simulink model "gm_uz_pmsm_model_9ph_dq"  (R2021b)
settings: Solver=FixedStepAuto  StartTime=0.0  StopTime=0.8  RelTol=1e-3
undefined symbols (not defined in the file or in its folder): c, friction_coefficient, inertia, k_i_d, k_i_q, k_p_d, k_p_q, Kpd, L_d, L_q, L_x1, L_x2, L_x3, L_y1, L_y2, L_y3, L_zero, polepair, psi_pm, R_1, static_friction_torque, Tnd
libraries: hdlmdlgenlib x137, dspsigops x19, slpidlib x2, pid_lib x1, spsdq0toAlphaBetaZeroLib x1
(part 1 of 2)
settings Model: Creator=ts  LastModifiedBy=valen
settings SolverCC: AlgebraicLoopSolver=TrustRegion  AutoInsertRateTranBlk=on
settings DataIOCC: LimitDataPoints=on  SaveOutput=off  SaveTime=off
settings OptimizationCC: BlockReduction=off  ConditionallyExecuteInputs=off  DefaultParameterBehavior=Inlined  InheritOutputTypeSmallerThanSingle=on  LifeSpan=inf
settings DebuggingCC: AlgebraicLoopMsg=error  InheritedTsInSrcMsg=none  SingleTaskRateTransMsg=error  AllowSymbolicDim=off  StrictBusMsg=ErrorOnBusTreatedAsVector  SFUnexpectedBacktrackingDiag=warning  SFNoUnconditionalDefaultTransitionDiag=warning  SFExecutionAtInitializationDiag=none  SFMachineParentedDataDiag=warning  ArithmeticOperatorsInVariantConditions=warning
settings HardwareCC: ProdBitPerPointer=32  ProdBitPerSizeT=32  ProdBitPerPtrDiffT=32  ProdLargestAtomicFloat=None  ProdIntDivRoundTo=Undefined  ProdEndianess=Unspecified  ProdWordSize=32  ProdHWDeviceType=ASIC/FPGA->ASIC/FPGA  ProdEqTarget=off
settings SFSimCC: SimUseLocalCustomCode=off  CustomCodeUndefinedFunction=UseInterfaceOnly
settings RTWCC: RTWUseLocalCustomCode=off
settings CodeAppCC: StateflowObjectComments=on
settings GRTTargetCC: TargetLangStandard=C89/C90 (ANSI)
settings ConfigComp: CovScope=ReferencedModels  CovMetricSettings=dw  CovSaveCumulativeToWorkspaceVar=on  CovSaveSingleToWorkspaceVar=on  CovExternalEMLEnable=off  CovSFcnEnable=off

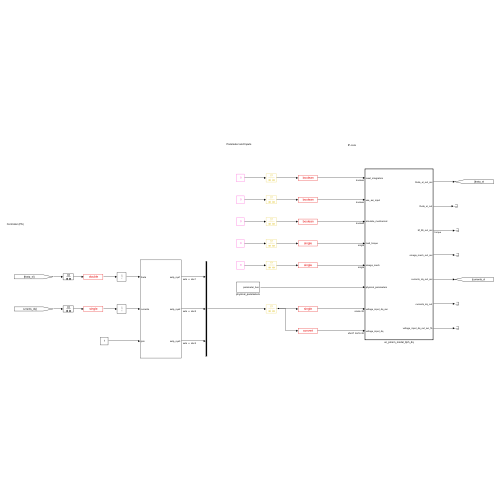
[thumbnail: Simulink's stored preview of the top-level diagram]
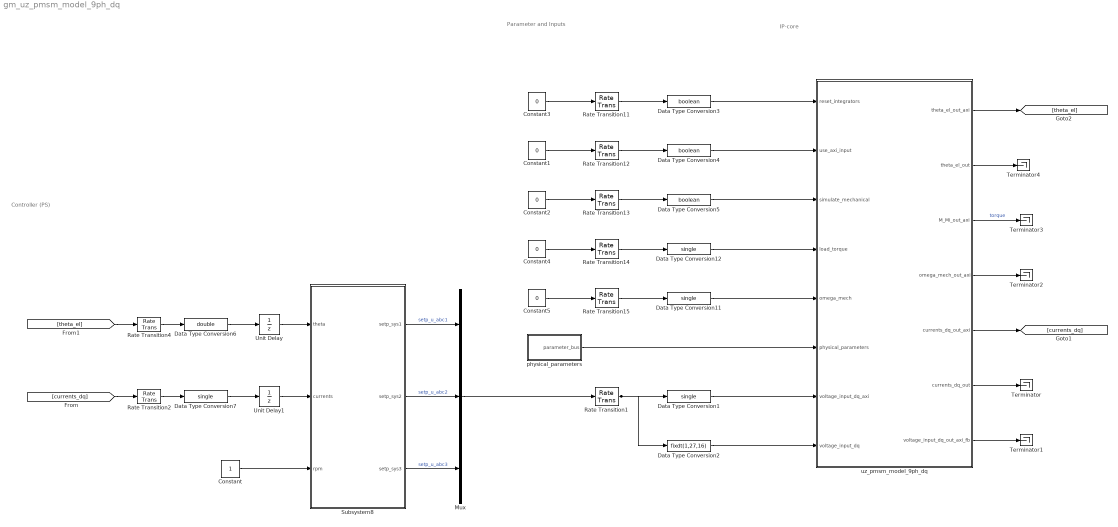
== system gm_uz_pmsm_model_9ph_dq ==
  note: IP-core
  note: Parameter and Inputs
  note: Controller (PS)
  Constant : Constant
  Constant{1..5} (5 alike) : Constant  Value=0
  Data Type Conversion{1,7,11..12} (4 alike) : DataTypeConversion  OutDataTypeStr=single
  Data Type Conversion2 : DataTypeConversion  OutDataTypeStr=fixdt(1,27,16)
  Data Type Conversion3 : DataTypeConversion  OutDataTypeStr=boolean
  Data Type Conversion4 : DataTypeConversion  OutDataTypeStr=boolean
  Data Type Conversion5 : DataTypeConversion  OutDataTypeStr=boolean
  Data Type Conversion6 : DataTypeConversion  OutDataTypeStr=double
  Mux : Mux  Inputs=3
  Rate Transition{1,11..15} (6 alike) : RateTransition  OutPortSampleTime=ts_pmsm
  Rate Transition2 : RateTransition  OutPortSampleTime=ts_isr
  Rate Transition4 : RateTransition  OutPortSampleTime=ts_isr
  Subsystem8 : Subsystem
  Terminator{,1..4} (5 alike) : Terminator
  Unit Delay : UnitDelay  SampleTime=-1  HasFrameUpgradeWarning=on
  Unit Delay1 : UnitDelay  SampleTime=-1  HasFrameUpgradeWarning=on
  physical_parameters : Subsystem
  uz_pmsm_model_9ph_dq : Subsystem  TreatAsAtomicUnit=on
  wires:
  Constant/1 -> Subsystem8/3(rpm)
  uz_pmsm_model_9ph_dq/2(theta_el_out) -> Terminator4/1
  uz_pmsm_model_9ph_dq/3(M_Mi_out_axi) -> Terminator3/1  "torque"
  uz_pmsm_model_9ph_dq/4(omega_mech_out_axi) -> Terminator2/1
  uz_pmsm_model_9ph_dq/7(voltage_input_dq_out_axi_fb) -> Terminator1/1
  uz_pmsm_model_9ph_dq/6(currents_dq_out) -> Terminator/1
  uz_pmsm_model_9ph_dq/5(currents_dq_out_axi) -> [currents_dq]
  uz_pmsm_model_9ph_dq/1(theta_el_out_axi) -> [theta_el]
  [currents_dq] -> Rate Transition2/1
  Data Type Conversion7/1 -> Unit Delay1/1
  Rate Transition2/1 -> Data Type Conversion7/1
  Unit Delay1/1 -> Subsystem8/2(currents)
  Unit Delay/1 -> Subsystem8/1(theta)
  Mux/1 -> Rate Transition1/1
  Data Type Conversion2/1 -> uz_pmsm_model_9ph_dq/8(voltage_input_dq)
  Data Type Conversion1/1 -> uz_pmsm_model_9ph_dq/7(voltage_input_dq_axi)
  Rate Transition1/1 -> Data Type Conversion1/1, Data Type Conversion2/1
  Subsystem8/1(setp_sys1) -> Mux/1  "setp_u_abc1"
  Subsystem8/2(setp_sys2) -> Mux/2  "setp_u_abc2"
  Subsystem8/3(setp_sys3) -> Mux/3  "setp_u_abc3"
  physical_parameters/1(parameter_bus) -> uz_pmsm_model_9ph_dq/6(physical_parameters)
  Constant4/1 -> Rate Transition14/1
  Constant5/1 -> Rate Transition15/1
  Data Type Conversion11/1 -> uz_pmsm_model_9ph_dq/5(omega_mech)
  Data Type Conversion12/1 -> uz_pmsm_model_9ph_dq/4(load_torque)
  Rate Transition14/1 -> Data Type Conversion12/1
  Rate Transition15/1 -> Data Type Conversion11/1
  Data Type Conversion5/1 -> uz_pmsm_model_9ph_dq/3(simulate_mechanical)
  Rate Transition13/1 -> Data Type Conversion5/1
  Constant2/1 -> Rate Transition13/1
  Constant1/1 -> Rate Transition12/1
  Rate Transition12/1 -> Data Type Conversion4/1
  Data Type Conversion4/1 -> uz_pmsm_model_9ph_dq/2(use_axi_input)
  Data Type Conversion3/1 -> uz_pmsm_model_9ph_dq/1(reset_integrators)
  Rate Transition11/1 -> Data Type Conversion3/1
  Constant3/1 -> Rate Transition11/1
  Rate Transition4/1 -> Data Type Conversion6/1
  Data Type Conversion6/1 -> Unit Delay/1
  [theta_el] -> Rate Transition4/1

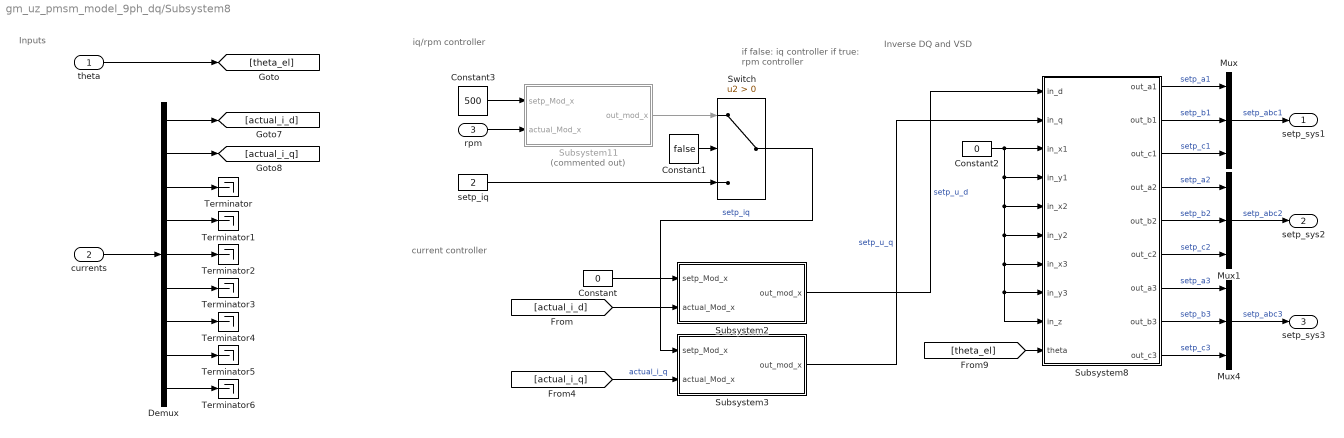
== system gm_uz_pmsm_model_9ph_dq/Subsystem8 ==
  note: Inverse DQ and VSD
  note: if false: iq controller
      | if true: rpm controller
  note: iq/rpm controller
  note: current controller
  note: Inputs
  theta : Inport
  currents : Inport  Port=2
  rpm : Inport  Port=3
  Constant : Constant  Value=0
  Constant1 : Constant  Value=false
  Constant2 : Constant  Value=0
  Constant3 : Constant  Value=500
  Demux : Demux  Outputs=9
  Mux : Mux  Inputs=3
  Mux1 : Mux  Inputs=3
  Mux4 : Mux  Inputs=3
  Subsystem11 : Subsystem  Commented=on
  Subsystem2 : Subsystem
  Subsystem3 : Subsystem
  Subsystem8 : Subsystem
  Switch : Switch  Criteria=u2 > Threshold
  Terminator{,1..6} (7 alike) : Terminator
  setp_iq : Constant  Value=2
  setp_sys1 : Outport
  setp_sys2 : Outport  Port=2
  setp_sys3 : Outport  Port=3
  wires:
  Demux/9 -> Terminator6/1
  Demux/6 -> Terminator3/1
  Demux/7 -> Terminator4/1
  Demux/8 -> Terminator5/1
  Demux/5 -> Terminator2/1
  Demux/4 -> Terminator1/1
  Demux/3 -> Terminator/1
  Demux/2 -> [actual_i_q]
  Demux/1 -> [actual_i_d]
  currents/1 -> Demux/1
  Subsystem2/1(out_mod_x) -> Subsystem8/1(in_d)  "setp_u_d"
  Subsystem3/1(out_mod_x) -> Subsystem8/2(in_q)  "setp_u_q"
  Constant3/1 -> Subsystem11/1(setp_Mod_x)
  setp_iq/1 -> Switch/3
  Constant1/1 -> Switch/2
  Switch/1 -> Subsystem3/1(setp_Mod_x)  "setp_iq"
  Subsystem11/1(out_mod_x) -> Switch/1
  Constant2/1 -> Subsystem8/4(in_y1), Subsystem8/5(in_x2), Subsystem8/6(in_y2), Subsystem8/7(in_x3), Subsystem8/9(in_z), Subsystem8/8(in_y3), Subsystem8/3(in_x1)
  rpm/1 -> Subsystem11/2(actual_Mod_x)
  Subsystem8/9(out_c3) -> Mux4/3  "setp_c3"
  Subsystem8/8(out_b3) -> Mux4/2  "setp_b3"
  Subsystem8/7(out_a3) -> Mux4/1  "setp_a3"
  Mux4/1 -> setp_sys3/1  "setp_abc3"
  Subsystem8/4(out_a2) -> Mux1/1  "setp_a2"
  Subsystem8/5(out_b2) -> Mux1/2  "setp_b2"
  Subsystem8/6(out_c2) -> Mux1/3  "setp_c2"
  Mux1/1 -> setp_sys2/1  "setp_abc2"
  Mux/1 -> setp_sys1/1  "setp_abc1"
  theta/1 -> [theta_el]
  [actual_i_q] -> Subsystem3/2(actual_Mod_x)  "actual_i_q"
  Constant/1 -> Subsystem2/1(setp_Mod_x)
  [actual_i_d] -> Subsystem2/2(actual_Mod_x)
  Subsystem8/3(out_c1) -> Mux/3  "setp_c1"
  Subsystem8/2(out_b1) -> Mux/2  "setp_b1"
  [theta_el] -> Subsystem8/10(theta)
  Subsystem8/1(out_a1) -> Mux/1  "setp_a1"

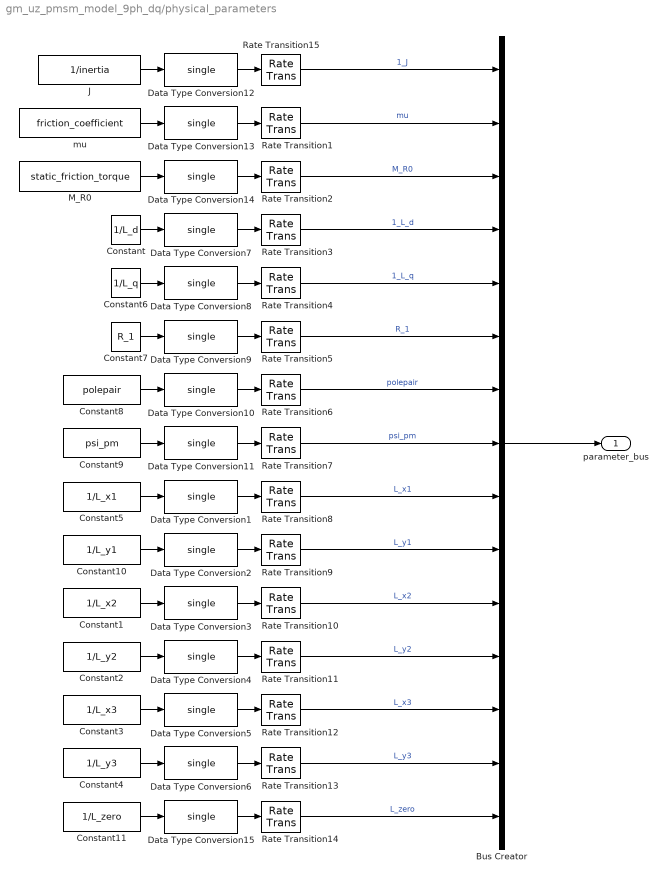
== system gm_uz_pmsm_model_9ph_dq/physical_parameters ==
  Bus Creator : BusCreator  Inputs=15
  Constant : Constant  Value=1/L_d
  Constant1 : Constant  Value=1/L_x2
  Constant10 : Constant  Value=1/L_y1
  Constant11 : Constant  Value=1/L_zero
  Constant2 : Constant  Value=1/L_y2
  Constant3 : Constant  Value=1/L_x3
  Constant4 : Constant  Value=1/L_y3
  Constant5 : Constant  Value=1/L_x1
  Constant6 : Constant  Value=1/L_q
  Constant7 : Constant  Value=R_1
  Constant8 : Constant  Value=polepair
  Constant9 : Constant  Value=psi_pm
  Data Type Conversion{1..15} (15 alike) : DataTypeConversion  OutDataTypeStr=single
  J : Constant  Value=1/inertia
  M_R0 : Constant  Value=static_friction_torque
  Rate Transition{1..15} (15 alike) : RateTransition  OutPortSampleTime=ts_pmsm
  mu : Constant  Value=friction_coefficient
  parameter_bus : Outport
  wires:
  Constant10/1 -> Data Type Conversion2/1
  Constant5/1 -> Data Type Conversion1/1
  Constant1/1 -> Data Type Conversion3/1
  Constant2/1 -> Data Type Conversion4/1
  Constant3/1 -> Data Type Conversion5/1
  Constant4/1 -> Data Type Conversion6/1
  Rate Transition9/1 -> Bus Creator/10  "L_y1"
  Rate Transition10/1 -> Bus Creator/11  "L_x2"
  Rate Transition11/1 -> Bus Creator/12  "L_y2"
  Rate Transition12/1 -> Bus Creator/13  "L_x3"
  Rate Transition13/1 -> Bus Creator/14  "L_y3"
  Rate Transition14/1 -> Bus Creator/15  "L_zero"
  Rate Transition8/1 -> Bus Creator/9  "L_x1"
  Data Type Conversion15/1 -> Rate Transition14/1
  Constant11/1 -> Data Type Conversion15/1
  Data Type Conversion6/1 -> Rate Transition13/1
  Data Type Conversion5/1 -> Rate Transition12/1
  Data Type Conversion4/1 -> Rate Transition11/1
  Data Type Conversion3/1 -> Rate Transition10/1
  Data Type Conversion2/1 -> Rate Transition9/1
  Data Type Conversion1/1 -> Rate Transition8/1
  Constant/1 -> Data Type Conversion7/1
  Constant9/1 -> Data Type Conversion11/1
  Constant7/1 -> Data Type Conversion9/1
  Data Type Conversion13/1 -> Rate Transition1/1
  Rate Transition4/1 -> Bus Creator/5  "1_L_q"
  M_R0/1 -> Data Type Conversion14/1
  mu/1 -> Data Type Conversion13/1
  Data Type Conversion10/1 -> Rate Transition6/1
  Data Type Conversion8/1 -> Rate Transition4/1
  J/1 -> Data Type Conversion12/1
  Rate Transition3/1 -> Bus Creator/4  "1_L_d"
  Constant6/1 -> Data Type Conversion8/1
  Rate Transition1/1 -> Bus Creator/2  "mu"
  Data Type Conversion9/1 -> Rate Transition5/1
  Constant8/1 -> Data Type Conversion10/1
  Data Type Conversion11/1 -> Rate Transition7/1
  Bus Creator/1 -> parameter_bus/1
  Rate Transition6/1 -> Bus Creator/7  "polepair"
  Rate Transition15/1 -> Bus Creator/1  "1_J"
  Rate Transition5/1 -> Bus Creator/6  "R_1"
  Data Type Conversion14/1 -> Rate Transition2/1
  Rate Transition7/1 -> Bus Creator/8  "psi_pm"
  Rate Transition2/1 -> Bus Creator/3  "M_R0"
  Data Type Conversion7/1 -> Rate Transition3/1
  Data Type Conversion12/1 -> Rate Transition15/1

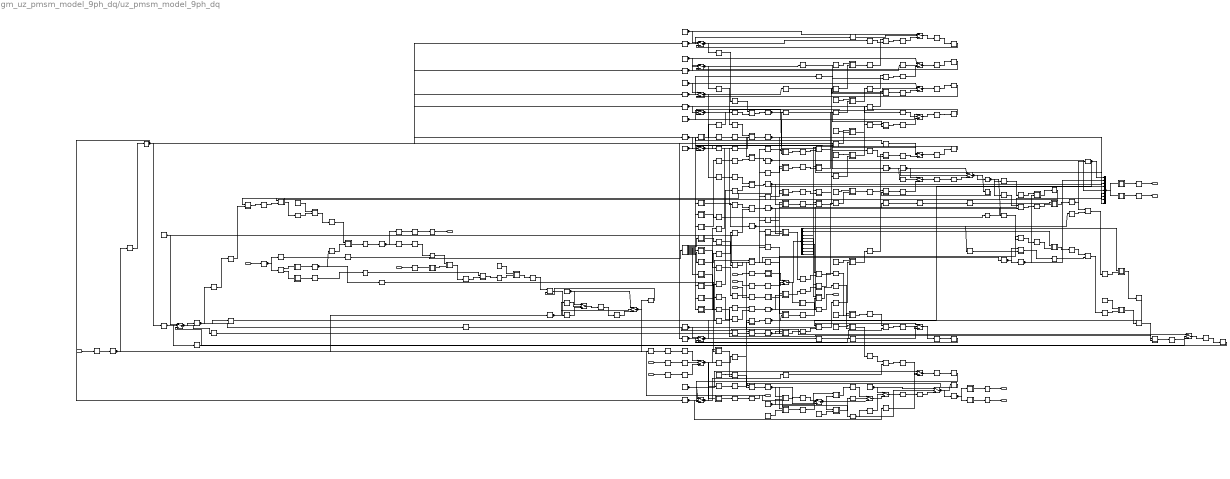
== system gm_uz_pmsm_model_9ph_dq/uz_pmsm_model_9ph_dq ==
  note: https://de.mathworks.com/help/releases/R2021a/hdlcoder/ug/troubleshoot-generate-implementation-model-from-simscape-pmsm.html?searchHighlight=troubleshoot-generate-implementation-model-from-simscape-pmsm&s_tid=doc_srchtitle
  note: load torque negative!!!
  note: zero equation
  note: y2 equation
  note: x2 equation
  note: y1 equation
  note: x1 equation
  note: o2 equation
  note: DQ equations
  note: o1 equation
  note: Inputs
  note: Mechanical and output
  note: PMSM electric and magentic
  note: This signal introduces an algebraic loop if simulate_mechanical is true!
  note: Input
  reset_integrators : Inport  OutDataTypeStr=boolean  PortDimensions=1  SampleTime=1e-06
  use_axi_input : Inport  Port=2  OutDataTypeStr=boolean  PortDimensions=1  SampleTime=1e-06
  simulate_mechanical : Inport  Port=3  OutDataTypeStr=boolean  PortDimensions=1  SampleTime=1e-06
  load_torque : Inport  Port=4  OutDataTypeStr=single  PortDimensions=1  SampleTime=1e-06
  omega_mech : Inport  Port=5  OutDataTypeStr=single  PortDimensions=1  SampleTime=1e-06
  physical_parameters : Inport  Port=6  SampleTime=1e-06
  voltage_input_dq_axi : Inport  Port=7  OutDataTypeStr=single  PortDimensions=[9]  SampleTime=1e-06
  voltage_input_dq : Inport  Port=8  OutDataTypeStr=fixdt(1, 27, 16)  PortDimensions=[9]  SampleTime=1e-06
  Add : Subsystem
      mask Display: disp('NFP\nadd');
  Add1 : Subsystem
      mask Display: disp('NFP\nadd');
  Add1_outbuff : hdlmdlgenlib/Buffer
      settings: SourceProductBaseCode=SL
  Add2 : Subsystem
      mask Display: disp('NFP\nadd');
  Add2_outbuff : hdlmdlgenlib/Buffer
      settings: SourceProductBaseCode=SL
  Add3 : Subsystem
      mask Display: disp('NFP\nadd');
  Add3_outbuff : hdlmdlgenlib/Buffer
      settings: SourceProductBaseCode=SL
  Add4 : Subsystem
      mask Display: disp('NFP\nadd');
  Add4_outbuff : hdlmdlgenlib/Buffer
      settings: SourceProductBaseCode=SL
  Add5 : Subsystem
      mask Display: disp('NFP\nadd');
  Add5_outbuff : hdlmdlgenlib/Buffer
      settings: SourceProductBaseCode=SL
  Add6 : Subsystem
      mask Display: disp('NFP\nadd');
  Add6_outbuff : hdlmdlgenlib/Buffer
      settings: SourceProductBaseCode=SL
  Add_outbuff : hdlmdlgenlib/Buffer
      settings: SourceProductBaseCode=SL
  Compare To Constant1_const : Constant  Value=double(-3.1415927410125732)  OutDataTypeStr=double  SampleTime=1e-08
  Compare To Constant1_relop : Subsystem
      mask Display: disp('NFP\nrelop');
  Compare To Constant1_relop_outbuff : hdlmdlgenlib/Buffer
      settings: SourceProductBaseCode=SL
  Compare To Constant_const : Constant  Value=double(3.1415927410125732)  OutDataTypeStr=double  SampleTime=1e-08
  Compare To Constant_relop : Subsystem
      mask Display: disp('NFP\nrelop');
  Compare To Constant_relop_outbuff : hdlmdlgenlib/Buffer
      settings: SourceProductBaseCode=SL
  Constant : Constant  Value=double(6.283185307179586)  OutDataTypeStr=double  SampleTime=1e-08
  Data Type Conversion1 : Subsystem
      mask Display: disp('NFP\nconv');
  Data Type Conversion10 : Subsystem
      mask Display: disp('NFP\nconv');
  Data Type Conversion101 : Subsystem
      mask Display: disp('NFP\nconv');
  Data Type Conversion11 : Subsystem
      mask Display: disp('NFP\nconv');
  Data Type Conversion111 : Subsystem
      mask Display: disp('NFP\nconv');
  Data Type Conversion12 : Subsystem
      mask Display: disp('NFP\nconv');
  Data Type Conversion121 : Subsystem
      mask Display: disp('NFP\nconv');
  Data Type Conversion13 : Subsystem
      mask Display: disp('NFP\nconv');
  Data Type Conversion14 : Subsystem
      mask Display: disp('NFP\nconv');
  Data Type Conversion15 : Subsystem
      mask Display: disp('NFP\nconv');
  Data Type Conversion2 : Subsystem
      mask Display: disp('NFP\nconv');
  Data Type Conversion21 : Subsystem
      mask Display: disp('NFP\nconv');
  Data Type Conversion3 : Subsystem
      mask Display: disp('NFP\nconv');
  Data Type Conversion31 : Subsystem
      mask Display: disp('NFP\nconv');
  Data Type Conversion4 : Subsystem
      mask Display: disp('NFP\nconv');
  Data Type Conversion41 : Subsystem
      mask Display: disp('NFP\nconv');
  Data Type Conversion5 : Subsystem
      mask Display: disp('NFP\nconv');
  Data Type Conversion51 : Subsystem
      mask Display: disp('NFP\nconv');
  Data Type Conversion6 : Subsystem
      mask Display: disp('NFP\nconv');
  Data Type Conversion61 : Subsystem
      mask Display: disp('NFP\nconv');
  Data Type Conversion7 : Subsystem
      mask Display: disp('NFP\nconv');
  Data Type Conversion71 : Subsystem
      mask Display: disp('NFP\nconv');
  Data Type Conversion8 : Subsystem
      mask Display: disp('NFP\nconv');
  Data Type Conversion81 : Subsystem
      mask Display: disp('NFP\nconv');
  Data Type Conversion9 : Subsystem
      mask Display: disp('NFP\nconv');
  Delay : RateTransition  OutPortSampleTimeOpt=Multiple of input port sample time  OutPortSampleTimeMultiple=100
  Delay1 : RateTransition  OutPortSampleTimeOpt=Multiple of input port sample time  OutPortSampleTimeMultiple=100
  Delay1_lowered{,1..10} (11 alike) : RateTransition  OutPortSampleTimeOpt=Multiple of input port sample time  OutPortSampleTimeMultiple=100
  Delay2 : RateTransition  OutPortSampleTimeOpt=Multiple of input port sample time  OutPortSampleTimeMultiple=100
  Divide : Subsystem
      mask Display: disp('NFP\nmul');
  Divide1 : Subsystem
      mask Display: disp('NFP\nmul');
  Divide10 : Subsystem
      mask Display: disp('NFP\nmul');
  Divide10_outbuff : hdlmdlgenlib/Buffer
      settings: SourceProductBaseCode=SL
  Divide11 : Subsystem
      mask Display: disp('NFP\nmul');
  Divide11_outbuff : hdlmdlgenlib/Buffer
      settings: SourceProductBaseCode=SL
  Divide12 : Subsystem
      mask Display: disp('NFP\nmul');
  Divide12_outbuff : hdlmdlgenlib/Buffer
      settings: SourceProductBaseCode=SL
  Divide13 : Subsystem
      mask Display: disp('NFP\nmul');
  Divide13_outbuff : hdlmdlgenlib/Buffer
      settings: SourceProductBaseCode=SL
  Divide1_outbuff : hdlmdlgenlib/Buffer
      settings: SourceProductBaseCode=SL
  Divide2 : Subsystem
      mask Display: disp('NFP\nmul');
  Divide2_outbuff : hdlmdlgenlib/Buffer
      settings: SourceProductBaseCode=SL
  Divide3 : Subsystem
      mask Display: disp('NFP\nmul');
  Divide3_outbuff : hdlmdlgenlib/Buffer
      settings: SourceProductBaseCode=SL
  Divide4 : Subsystem
      mask Display: disp('NFP\nmul');
  Divide4_outbuff : hdlmdlgenlib/Buffer
      settings: SourceProductBaseCode=SL
  Divide5 : Subsystem
      mask Display: disp('NFP\nmul');
  Divide5_outbuff : hdlmdlgenlib/Buffer
      settings: SourceProductBaseCode=SL
  Divide6 : Subsystem
      mask Display: disp('NFP\nmul');
  Divide6_outbuff : hdlmdlgenlib/Buffer
      settings: SourceProductBaseCode=SL
  Divide7 : Subsystem
      mask Display: disp('NFP\nmul');
  Divide7_outbuff : hdlmdlgenlib/Buffer
      settings: SourceProductBaseCode=SL
  Divide8 : Subsystem
      mask Display: disp('NFP\nmul');
  Divide8_outbuff : hdlmdlgenlib/Buffer
      settings: SourceProductBaseCode=SL
  Divide9 : Subsystem
      mask Display: disp('NFP\nmul');
  Divide9_outbuff : hdlmdlgenlib/Buffer
      settings: SourceProductBaseCode=SL
  Divide_outbuff : hdlmdlgenlib/Buffer
      settings: SourceProductBaseCode=SL
  Factor : Subsystem
      mask Display: disp('NFP\nmul');
  Factor_const : Constant  Value=double(4.5)  OutDataTypeStr=double  SampleTime=1e-08
  Factor_outbuff : hdlmdlgenlib/Buffer
      settings: SourceProductBaseCode=SL
  From{,1..27,30..32,41,51,61,71,91,121} (37 alike) : hdlmdlgenlib/Buffer
      settings: SourceProductBaseCode=SL
  Gain : Subsystem
      mask Display: disp('NFP\nmul');
  Gain1 : Subsystem
      mask Display: disp('NFP\nmul');
  Gain10 : Subsystem
      mask Display: disp('NFP\nmul');
  Gain2 : Subsystem
      mask Display: disp('NFP\nmul');
  Gain3 : Subsystem
      mask Display: disp('NFP\nmul');
  Gain4 : Subsystem
      mask Display: disp('NFP\nmul');
  Gain5 : Subsystem
      mask Display: disp('NFP\nmul');
  Gain6 : Subsystem
      mask Display: disp('NFP\nmul');
  Gain7 : Subsystem
      mask Display: disp('NFP\nmul');
  Gain8 : Subsystem
      mask Display: disp('NFP\nmul');
  Gain9 : Subsystem
      mask Display: disp('NFP\nmul');
  Gain_const{,1..10} (11 alike) : Constant  Value=double(1e-06)  OutDataTypeStr=double  SampleTime=1e-08
  Gain_outbuff{,1..9} (10 alike) : hdlmdlgenlib/Buffer
      settings: SourceProductBaseCode=SL
  Goto{1..4,9..16,32..36,361} (18 alike) : hdlmdlgenlib/Buffer
      settings: SourceProductBaseCode=SL
  Initial_Val{,1..10} (11 alike) : Constant  Value=double(0)  OutDataTypeStr=double  SampleTime=1e-08
  M_Mi : hdlmdlgenlib/Buffer
      settings: SourceProductBaseCode=SL
  Product : Subsystem
      mask Display: disp('NFP\nmul');
  Product1 : Subsystem
      mask Display: disp('NFP\nmul');
  Product10 : Subsystem
      mask Display: disp('NFP\nmul');
  Product10_outbuff : hdlmdlgenlib/Buffer
      settings: SourceProductBaseCode=SL
  Product11 : Subsystem
      mask Display: disp('NFP\nmul');
  Product11_outbuff : hdlmdlgenlib/Buffer
      settings: SourceProductBaseCode=SL
  Product1_outbuff : hdlmdlgenlib/Buffer
      settings: SourceProductBaseCode=SL
  Product2 : Subsystem
      mask Display: disp('NFP\nmul');
  Product21 : Subsystem
      mask Display: disp('NFP\nmul');
  Product2_outbuff : hdlmdlgenlib/Buffer
      settings: SourceProductBaseCode=SL
  Product3 : Subsystem
      mask Display: disp('NFP\nmul');
  Product3_outbuff : hdlmdlgenlib/Buffer
      settings: SourceProductBaseCode=SL
  Product5 : Subsystem
      mask Display: disp('NFP\nmul');
  Product5_outbuff : hdlmdlgenlib/Buffer
      settings: SourceProductBaseCode=SL
  Product6 : Subsystem
      mask Display: disp('NFP\nmul');
  Product6_outbuff : hdlmdlgenlib/Buffer
      settings: SourceProductBaseCode=SL
  Product7 : Subsystem
      mask Display: disp('NFP\nmul');
  Product7_outbuff : hdlmdlgenlib/Buffer
      settings: SourceProductBaseCode=SL
  Product8 : Subsystem
      mask Display: disp('NFP\nmul');
  Product8_outbuff : hdlmdlgenlib/Buffer
      settings: SourceProductBaseCode=SL
  Product9 : Subsystem
      mask Display: disp('NFP\nmul');
  Product9_outbuff : hdlmdlgenlib/Buffer
      settings: SourceProductBaseCode=SL
  Product_outbuff : hdlmdlgenlib/Buffer
      settings: SourceProductBaseCode=SL
  Sum : Subsystem
      mask Display: disp('NFP\nadd');
  Sum1 : Subsystem
      mask Display: disp('NFP\nadd');
  Sum11 : Subsystem
      mask Display: disp('NFP\nadd');
  Sum1_outbuff : hdlmdlgenlib/Buffer
      settings: SourceProductBaseCode=SL
  Sum1_outbuff1 : hdlmdlgenlib/Buffer
      settings: SourceProductBaseCode=SL
  Sum1_stage2 : Subsystem
      mask Display: disp('NFP\nadd');
  Sum1_stage2_outbuff : hdlmdlgenlib/Buffer
      settings: SourceProductBaseCode=SL
  Sum1_stage3 : Subsystem
      mask Display: disp('NFP\nadd');
  Sum1_stage3_outbuff : hdlmdlgenlib/Buffer
      settings: SourceProductBaseCode=SL
  Sum2 : Subsystem
      mask Display: disp('NFP\nadd');
  Sum21 : Subsystem
      mask Display: disp('NFP\nadd');
  Sum2_outbuff : hdlmdlgenlib/Buffer
      settings: SourceProductBaseCode=SL
  Sum2_outbuff1 : hdlmdlgenlib/Buffer
      settings: SourceProductBaseCode=SL
  Sum3 : Subsystem
      mask Display: disp('NFP\nadd');
  Sum31 : Subsystem
      mask Display: disp('NFP\nadd');
  Sum310 : Subsystem
      mask Display: disp('NFP\nadd');
  Sum32 : Subsystem
      mask Display: disp('NFP\nadd');
  Sum33 : Subsystem
      mask Display: disp('NFP\nadd');
  Sum34 : Subsystem
      mask Display: disp('NFP\nadd');
  Sum35 : Subsystem
      mask Display: disp('NFP\nadd');
  Sum36 : Subsystem
      mask Display: disp('NFP\nadd');
  Sum37 : Subsystem
      mask Display: disp('NFP\nadd');
  Sum38 : Subsystem
      mask Display: disp('NFP\nadd');
  Sum39 : Subsystem
      mask Display: disp('NFP\nadd');
  Sum3_outbuff{,1..10} (11 alike) : hdlmdlgenlib/Buffer
      settings: SourceProductBaseCode=SL
  Sum_outbuff : hdlmdlgenlib/Buffer
      settings: SourceProductBaseCode=SL
  Sum_stage2 : Subsystem
      mask Display: disp('NFP\nadd');
  Sum_stage2_outbuff : hdlmdlgenlib/Buffer
      settings: SourceProductBaseCode=SL
  Sum_stage3 : Subsystem
      mask Display: disp('NFP\nadd');
  Sum_stage3_outbuff : hdlmdlgenlib/Buffer
      settings: SourceProductBaseCode=SL
  Switch{,1..2,11} (4 alike) : Switch  Criteria=u2 ~= 0  Threshold=double(0)  OutDataTypeStr=double  SampleTime=1e-08
  bus_selector : BusSelector  OutputSignals=1_L_d,1_L_q,R_1,polepair,psi_pm,L_x1,L_y1,L_x2,L_y2,L_x3,L_y3,L_zero
  bus_selector1 : BusSelector  OutputSignals=polepair,1_J
  delayMatch{,1..38} (39 alike) : Delay  DelayLength=double(1)  InitialCondition=0  SampleTime=1e-08
  delayMatch39 : Delay  DelayLength=double(1)  InitialCondition=0  SampleTime=1e-06
  delayMatch40 : Delay  DelayLength=double(1)  InitialCondition=0  SampleTime=1e-06
  i_d : hdlmdlgenlib/Buffer
      settings: SourceProductBaseCode=SL
  i_q : hdlmdlgenlib/Buffer
      settings: SourceProductBaseCode=SL
  in0_repeat : dspsigops/Repeat  N=double(100)  RateOptions=Allow multirate processing  ic=0  mode=Unused parameter value
  in10_repeat : dspsigops/Repeat  N=double(100)  RateOptions=Allow multirate processing  ic=0  mode=Unused parameter value
  in11_repeat : dspsigops/Repeat  N=double(100)  RateOptions=Allow multirate processing  ic=0  mode=Unused parameter value
  in12_repeat : dspsigops/Repeat  N=double(100)  RateOptions=Allow multirate processing  ic=0  mode=Unused parameter value
  in13_repeat : RateTransition  Integrity=off  Deterministic=off  OutPortSampleTimeOpt=Multiple of input port sample time  OutPortSampleTimeMultiple=1/100
  in14_repeat : dspsigops/Repeat  N=double(100)  RateOptions=Allow multirate processing  ic=0  mode=Unused parameter value
  in15_repeat : dspsigops/Repeat  N=double(100)  RateOptions=Allow multirate processing  ic=0  mode=Unused parameter value
  in16_repeat : dspsigops/Repeat  N=double(100)  RateOptions=Allow multirate processing  ic=0  mode=Unused parameter value
  in17_repeat : dspsigops/Repeat  N=double(100)  RateOptions=Allow multirate processing  ic=0  mode=Unused parameter value
  in18_repeat : dspsigops/Repeat  N=double(100)  RateOptions=Allow multirate processing  ic=0  mode=Unused parameter value
  in19_repeat : dspsigops/Repeat  N=double(100)  RateOptions=Allow multirate processing  ic=0  mode=Unused parameter value
  in1_repeat : dspsigops/Repeat  N=double(100)  RateOptions=Allow multirate processing  ic=0  mode=Unused parameter value
  in2_repeat : dspsigops/Repeat  N=double(100)  RateOptions=Allow multirate processing  ic=0  mode=Unused parameter value
  in3_repeat : dspsigops/Repeat  N=double(100)  RateOptions=Allow multirate processing  ic=0  mode=Unused parameter value
  in4_repeat : dspsigops/Repeat  N=double(100)  RateOptions=Allow multirate processing  ic=0  mode=Unused parameter value
  in5_repeat : dspsigops/Repeat  N=double(100)  RateOptions=Allow multirate processing  ic=0  mode=Unused parameter value
  in6_repeat : dspsigops/Repeat  N=double(100)  RateOptions=Allow multirate processing  ic=0  mode=Unused parameter value
  in7_repeat : dspsigops/Repeat  N=double(100)  RateOptions=Allow multirate processing  ic=0  mode=Unused parameter value
  in8_repeat : dspsigops/Repeat  N=double(100)  RateOptions=Allow multirate processing  ic=0  mode=Unused parameter value
  in9_repeat : dspsigops/Repeat  N=double(100)  RateOptions=Allow multirate processing  ic=0  mode=Unused parameter value
  integrator_out1 : hdlmdlgenlib/Buffer
      settings: SourceProductBaseCode=SL
  mechanical_system_out1 : hdlmdlgenlib/Buffer
      settings: SourceProductBaseCode=SL
  mux : Mux  Inputs=9
  pmsm_out1 : hdlmdlgenlib/Buffer
      settings: SourceProductBaseCode=SL
  pmsm_out2 : hdlmdlgenlib/Buffer
      settings: SourceProductBaseCode=SL
  psi_{,1..6} (7 alike) : hdlmdlgenlib/Buffer
      settings: SourceProductBaseCode=SL
  psi_d : hdlmdlgenlib/Buffer
      settings: SourceProductBaseCode=SL
  psi_q : hdlmdlgenlib/Buffer
      settings: SourceProductBaseCode=SL
  reset_in{,1..10} (11 alike) : Switch  Criteria=u2 ~= 0  Threshold=double(0)  OutDataTypeStr=double  SampleTime=1e-08
  reset_out{,1..10} (11 alike) : Switch  Criteria=u2 ~= 0  Threshold=double(0)  OutDataTypeStr=double  SampleTime=1e-08
  t : Demux  Outputs=9
  t{1..5} (5 alike) : RateTransition  OutPortSampleTimeOpt=Multiple of input port sample time  OutPortSampleTimeMultiple=100
  theta_el : hdlmdlgenlib/Buffer
      settings: SourceProductBaseCode=SL
  theta_el_out_axi : Outport  SampleTime=1e-06
  theta_el_out : Outport  Port=2  SampleTime=1e-06
  M_Mi_out_axi : Outport  Port=3  SampleTime=1e-06
  omega_mech_out_axi : Outport  Port=4  SampleTime=1e-06
  currents_dq_out_axi : Outport  Port=5  SampleTime=1e-06
  currents_dq_out : Outport  Port=6  SampleTime=1e-06
  voltage_input_dq_out_axi_fb : Outport  Port=7  SampleTime=1e-06
  wires:
  reset_integrators/1 -> in3_repeat/1
  use_axi_input/1 -> in16_repeat/1
  simulate_mechanical/1 -> in5_repeat/1
  load_torque/1 -> in1_repeat/1
  omega_mech/1 -> in6_repeat/1
  physical_parameters/1 -> in13_repeat/1
  voltage_input_dq_axi/1 -> in15_repeat/1
  voltage_input_dq/1 -> in17_repeat/1
  delayMatch39/1 -> M_Mi_out_axi/1
  delayMatch40/1 -> omega_mech_out_axi/1
  t1/1 -> currents_dq_out/1
  t2/1 -> currents_dq_out_axi/1
  t3/1 -> theta_el_out/1
  t4/1 -> theta_el_out_axi/1
  t5/1 -> voltage_input_dq_out_axi_fb/1
  Delay1/1 -> delayMatch39/1
  Delay2/1 -> delayMatch40/1
  Delay/1 -> in0_repeat/1
  Delay1_lowered/1 -> in19_repeat/1
  Delay1_lowered1/1 -> in18_repeat/1
  Delay1_lowered2/1 -> in14_repeat/1
  Delay1_lowered3/1 -> in4_repeat/1
  Delay1_lowered4/1 -> in2_repeat/1
  Delay1_lowered5/1 -> in7_repeat/1
  Delay1_lowered6/1 -> in8_repeat/1
  Delay1_lowered7/1 -> in9_repeat/1
  Delay1_lowered8/1 -> in10_repeat/1
  Delay1_lowered9/1 -> in11_repeat/1
  Delay1_lowered10/1 -> in12_repeat/1
  M_Mi/1 -> Delay/1, Data Type Conversion14/1(In1)
  reset_in10/1 -> Delay1_lowered/1
  reset_in/1 -> Delay1_lowered1/1
  reset_in9/1 -> Delay1_lowered2/1
  reset_in2/1 -> Delay1_lowered3/1
  reset_in1/1 -> Delay1_lowered4/1
  reset_in3/1 -> Delay1_lowered5/1
  reset_in4/1 -> Delay1_lowered6/1
  reset_in5/1 -> Delay1_lowered7/1
  reset_in6/1 -> Delay1_lowered8/1
  reset_in7/1 -> Delay1_lowered9/1
  reset_in8/1 -> Delay1_lowered10/1
  in0_repeat/1 -> delayMatch24/1
  in1_repeat/1 -> Data Type Conversion7/1(In1)
  in2_repeat/1 -> reset_out/3
  in3_repeat/1 -> Goto3/1
  in4_repeat/1 -> reset_out1/3
  in5_repeat/1 -> delayMatch13/1
  in6_repeat/1 -> Data Type Conversion13/1(In1)
  in7_repeat/1 -> reset_out2/3
  in8_repeat/1 -> reset_out3/3
  in9_repeat/1 -> reset_out4/3
  in10_repeat/1 -> reset_out5/3
  in11_repeat/1 -> reset_out6/3
  in12_repeat/1 -> reset_out7/3
  in13_repeat/1 -> bus_selector1/1, Goto2/1
  in14_repeat/1 -> reset_out8/3
  in15_repeat/1 -> Data Type Conversion61/1(In1)
  in16_repeat/1 -> delayMatch11/1
  in17_repeat/1 -> Data Type Conversion101/1(In1)
  in18_repeat/1 -> reset_out9/3
  in19_repeat/1 -> reset_out10/3
  Initial_Val/1 -> reset_out9/1, reset_in/1
  Sum3_outbuff/1 -> reset_in/3
  Gain_outbuff/1 -> Sum3/1(In1)
  delayMatch3/1 -> Product21/2(In2)
  Product1_outbuff/1 -> Sum1_stage2/2(In2)
  theta_el/1 -> Data Type Conversion5/1(In1), Data Type Conversion12/1(In1)
  From6/1 -> Goto16/1
  delayMatch12/1 -> Switch11/1
  integrator_out1/1 -> mechanical_system_out1/1
  Initial_Val1/1 -> reset_out/1, reset_in1/1
  Goto1/1 -> From1/1
  Sum1_outbuff/1 -> Product11/2(In2)
  Product11_outbuff/1 -> Gain1/2(In2)
  Gain_outbuff1/1 -> Sum31/1(In1)
  Sum3_outbuff1/1 -> reset_in1/3
  delayMatch25/1 -> Sum31/2(In2)
  delayMatch26/1 -> reset_in1/2
  Goto3/1 -> From6/1, From3/1, From2/1
  delayMatch23/1 -> reset_in2/2
  delayMatch22/1 -> Sum/1(In1)
  Initial_Val2/1 -> reset_out1/1, reset_in2/1
  Switch1/1 -> reset_in2/3
  Sum1_outbuff1/1 -> Switch/1
  Constant/1 -> Sum2/1(In1), Sum11/2(In2)
  Sum2_outbuff/1 -> Switch1/1
  From/1 -> Product/2(In2)
  Switch11/1 -> Product/1(In1), Data Type Conversion4/1(In1), Goto4/1
  Goto4/1 -> From7/1
  From7/1 -> Product10/1(In1)
  Goto36/1 -> From10/1
  Goto9/1 -> From11/1
  From11/1 -> Divide1/2(In2)
  Divide1_outbuff/1 -> Divide/2(In2), mux/3
  delayMatch4/1 -> Divide1/1(In1)
  delayMatch28/1 -> reset_in3/2
  delayMatch27/1 -> Sum32/2(In2)
  Initial_Val3/1 -> reset_out2/1, reset_in3/1
  Sum3_outbuff2/1 -> reset_in3/3
  Gain_outbuff2/1 -> Sum32/1(In1)
  Add_outbuff/1 -> Gain3/2(In2)
  Divide_outbuff/1 -> Add/2(In2)
  Goto15/1 -> From21/1
  From21/1 -> Divide13/2(In2)
  Divide13_outbuff/1 -> Divide12/2(In2), mux/9
  delayMatch10/1 -> Divide13/1(In1)
  delayMatch30/1 -> reset_in4/2
  delayMatch29/1 -> Sum33/2(In2)
  Initial_Val4/1 -> reset_out3/1, reset_in4/1
  Sum3_outbuff3/1 -> reset_in4/3
  Gain_outbuff3/1 -> Sum33/1(In1)
  Add6_outbuff/1 -> Gain4/2(In2)
  Divide12_outbuff/1 -> Add6/2(In2)
  Goto14/1 -> From20/1
  From20/1 -> Divide11/2(In2)
  Divide11_outbuff/1 -> Divide10/2(In2), mux/8
  delayMatch9/1 -> Divide11/1(In1)
  delayMatch32/1 -> reset_in5/2
  delayMatch31/1 -> Sum34/2(In2)
  Initial_Val5/1 -> reset_out4/1, reset_in5/1
  Sum3_outbuff4/1 -> reset_in5/3
  Gain_outbuff4/1 -> Sum34/1(In1)
  Add5_outbuff/1 -> Gain5/2(In2)
  Divide10_outbuff/1 -> Add5/2(In2)
  Goto13/1 -> From17/1
  From17/1 -> Divide9/2(In2)
  Divide9_outbuff/1 -> Divide8/2(In2), mux/7
  delayMatch8/1 -> Divide9/1(In1)
  delayMatch34/1 -> reset_in6/2
  delayMatch33/1 -> Sum35/2(In2)
  Initial_Val6/1 -> reset_out5/1, reset_in6/1
  Sum3_outbuff5/1 -> reset_in6/3
  Gain_outbuff5/1 -> Sum35/1(In1)
  Add4_outbuff/1 -> Gain6/2(In2)
  Divide8_outbuff/1 -> Add4/2(In2)
  Goto12/1 -> From16/1
  From16/1 -> Divide7/2(In2)
  Divide7_outbuff/1 -> Divide6/2(In2), mux/6
  delayMatch7/1 -> Divide7/1(In1)
  delayMatch36/1 -> reset_in7/2
  delayMatch35/1 -> Sum36/2(In2)
  Initial_Val7/1 -> reset_out6/1, reset_in7/1
  Sum3_outbuff6/1 -> reset_in7/3
  Gain_outbuff6/1 -> Sum36/1(In1)
  Add3_outbuff/1 -> Gain7/2(In2)
  Divide6_outbuff/1 -> Add3/2(In2)
  Goto11/1 -> From13/1
  From13/1 -> Divide5/2(In2)
  Divide5_outbuff/1 -> Divide4/2(In2), mux/5
  delayMatch6/1 -> Divide5/1(In1)
  delayMatch38/1 -> reset_in8/2
  delayMatch37/1 -> Sum37/2(In2)
  Initial_Val8/1 -> reset_out7/1, reset_in8/1
  Sum3_outbuff7/1 -> reset_in8/3
  Gain_outbuff7/1 -> Sum37/1(In1)
  Add2_outbuff/1 -> Gain8/2(In2)
  Divide4_outbuff/1 -> Add2/2(In2)
  Goto32/1 -> From8/1, From4/1, From30/1, From26/1, From22/1, From18/1, From14/1, From12/1, From9/1
  Product6_outbuff/1 -> Product7/1(In1), i_q/1
  From71/1 -> Product6/2(In2)
  Goto35/1 -> From71/1
  From24/1 -> Sum21/2(In2)
  Goto33/1 -> From24/1
  From121/1 -> Divide3/2(In2)
  Goto10/1 -> From121/1
  Goto2/1 -> From51/1
  From51/1 -> bus_selector/1
  bus_selector/1 -> Data Type Conversion6/1(In1)  "<1_L_d>"
  bus_selector/2 -> Data Type Conversion1/1(In1)  "<1_L_q>"
  bus_selector/3 -> Data Type Conversion21/1(In1)  "<R_1>"
  bus_selector/4 -> Data Type Conversion31/1(In1)  "<polepair>"
  bus_selector/5 -> Data Type Conversion41/1(In1)  "<psi_pm>"
  bus_selector/6 -> Data Type Conversion51/1(In1)  "<L_x1>"
  bus_selector/7 -> Data Type Conversion71/1(In1)  "<L_y1>"
  bus_selector/8 -> Data Type Conversion8/1(In1)  "<L_x2>"
  bus_selector/9 -> Data Type Conversion9/1(In1)  "<L_y2>"
  bus_selector/10 -> Data Type Conversion10/1(In1)  "<L_x3>"
  bus_selector/11 -> Data Type Conversion111/1(In1)  "<L_y3>"
  bus_selector/12 -> Data Type Conversion121/1(In1)  "<L_zero>"
  Goto34/1 -> From61/1
  From61/1 -> Product10/2(In2)
  Product10_outbuff/1 -> Product2/1(In1), Product1/1(In1)
  delayMatch/1 -> Product6/1(In1)
  delayMatch21/1 -> reset_in9/2
  delayMatch20/1 -> Sum38/2(In2)
  Initial_Val9/1 -> reset_out8/1, reset_in9/1
  Sum3_outbuff8/1 -> reset_in9/3
  Gain_outbuff8/1 -> Sum38/1(In1)
  Sum1_stage3_outbuff/1 -> Gain9/2(In2)
  Switch2/1 -> Data Type Conversion81/1(In1), t/1
  Add1_outbuff/1 -> Gain/2(In2)
  Divide2_outbuff/1 -> Add1/2(In2)
  Divide3_outbuff/1 -> Divide2/2(In2), mux/4
  delayMatch5/1 -> Divide3/1(In1)
  delayMatch17/1 -> Sum3/2(In2)
  delayMatch18/1 -> reset_in/2
  Goto16/1 -> From91/1, From5/1, From31/1, From32/1, From27/1, From23/1, From25/1, From19/1, From15/1
  delayMatch16/1 -> reset_in10/2
  delayMatch15/1 -> Sum39/2(In2)
  Initial_Val10/1 -> reset_out10/1, reset_in10/1
  Sum3_outbuff9/1 -> reset_in10/3
  Gain_outbuff9/1 -> Sum39/1(In1)
  Sum_stage3_outbuff/1 -> Gain10/2(In2)
  Product8_outbuff/1 -> Sum_stage2/2(In2)
  Product5_outbuff/1 -> Product8/1(In1), i_d/1
  Sum2_outbuff1/1 -> Product5/2(In2)
  delayMatch1/1 -> Sum21/1(In1)
  delayMatch2/1 -> Product3/1(In1)
  mux/1 -> Data Type Conversion11/1(In1), Data Type Conversion3/1(In1)
  i_d/1 -> Product21/1(In1), mux/1
  Product2_outbuff/1 -> Sum310/2(In2)
  Sum3_outbuff10/1 -> Factor/2(In2)
  Factor_outbuff/1 -> Product9/1(In1)
  Product9_outbuff/1 -> M_Mi/1
  Goto361/1 -> From41/1, From/1
  bus_selector1/1 -> Data Type Conversion15/1(In1)  "<polepair>"
  bus_selector1/2 -> Data Type Conversion2/1(In1)  "<1_J>"
  Compare To Constant1_const/1 -> Compare To Constant1_relop/2(In2)
  Compare To Constant_const/1 -> Compare To Constant_relop/2(In2)
  Sum1_stage2_outbuff/1 -> Sum1_stage3/1(In1)
  t/1 -> Sum_stage2/1(In1)
  t/2 -> Sum1_stage2/1(In1)
  t/3 -> Add/1(In1)
  t/4 -> Add1/1(In1)
  t/5 -> Add2/1(In1)
  t/6 -> Add3/1(In1)
  t/7 -> Add4/1(In1)
  t/8 -> Add5/1(In1)
  t/9 -> Add6/1(In1)
  Sum_stage2_outbuff/1 -> Sum_stage3/1(In1)
  Gain_const/1 -> Gain/1(In1)
  Gain_const1/1 -> Gain1/1(In1)
  Gain_const2/1 -> Gain2/1(In1)
  Gain_const3/1 -> Gain3/1(In1)
  Gain_const4/1 -> Gain4/1(In1)
  Gain_const5/1 -> Gain5/1(In1)
  Gain_const6/1 -> Gain6/1(In1)
  Gain_const7/1 -> Gain7/1(In1)
  Gain_const8/1 -> Gain8/1(In1)
  Gain_const9/1 -> Gain9/1(In1)
  Gain_const10/1 -> Gain10/1(In1)
  Factor_const/1 -> Factor/1(In1)
  delayMatch24/1 -> Sum1/1(In1)
  delayMatch13/1 -> Switch11/2
  delayMatch11/1 -> Switch2/2
  Data Type Conversion14/1(Out1) -> Delay1/1
  Data Type Conversion3/1(Out1) -> t1/1
  Data Type Conversion11/1(Out1) -> t2/1
  Sum3/1(Out1) -> Sum3_outbuff/1
  Product1/1(Out1) -> Product1_outbuff/1
  Data Type Conversion4/1(Out1) -> Delay2/1
  Data Type Conversion12/1(Out1) -> t3/1
  Data Type Conversion5/1(Out1) -> t4/1
  Data Type Conversion2/1(Out1) -> Goto1/1
  Data Type Conversion7/1(Out1) -> Sum1/2(In2)
  Sum1/1(Out1) -> Sum1_outbuff/1
  Product11/1(Out1) -> Product11_outbuff/1
  Sum31/1(Out1) -> Sum3_outbuff1/1
  Compare To Constant1_relop/1(Out1) -> Compare To Constant1_relop_outbuff/1
  Sum11/1(Out1) -> Sum1_outbuff1/1
  Sum2/1(Out1) -> Sum2_outbuff/1
  Compare To Constant_relop/1(Out1) -> Compare To Constant_relop_outbuff/1
  Sum/1(Out1) -> Sum_outbuff/1
  Product/1(Out1) -> Gain2/2(In2)
  Data Type Conversion13/1(Out1) -> Switch11/3
  Data Type Conversion6/1(Out1) -> Goto36/1
  Data Type Conversion51/1(Out1) -> Goto9/1
  Divide1/1(Out1) -> Divide1_outbuff/1
  Sum32/1(Out1) -> Sum3_outbuff2/1
  Add/1(Out1) -> Add_outbuff/1
  Divide/1(Out1) -> Divide_outbuff/1
  Data Type Conversion121/1(Out1) -> Goto15/1
  Divide13/1(Out1) -> Divide13_outbuff/1
  Sum33/1(Out1) -> Sum3_outbuff3/1
  Add6/1(Out1) -> Add6_outbuff/1
  Divide12/1(Out1) -> Divide12_outbuff/1
  Data Type Conversion111/1(Out1) -> Goto14/1
  Divide11/1(Out1) -> Divide11_outbuff/1
  Sum34/1(Out1) -> Sum3_outbuff4/1
  Add5/1(Out1) -> Add5_outbuff/1
  Divide10/1(Out1) -> Divide10_outbuff/1
  Data Type Conversion10/1(Out1) -> Goto13/1
  Divide9/1(Out1) -> Divide9_outbuff/1
  Sum35/1(Out1) -> Sum3_outbuff5/1
  Add4/1(Out1) -> Add4_outbuff/1
  Divide8/1(Out1) -> Divide8_outbuff/1
  Data Type Conversion9/1(Out1) -> Goto12/1
  Divide7/1(Out1) -> Divide7_outbuff/1
  Sum36/1(Out1) -> Sum3_outbuff6/1
  Add3/1(Out1) -> Add3_outbuff/1
  Divide6/1(Out1) -> Divide6_outbuff/1
  Data Type Conversion8/1(Out1) -> Goto11/1
  Divide5/1(Out1) -> Divide5_outbuff/1
  Sum37/1(Out1) -> Sum3_outbuff7/1
  Add2/1(Out1) -> Add2_outbuff/1
  Divide4/1(Out1) -> Divide4_outbuff/1
  Data Type Conversion21/1(Out1) -> Goto32/1
  Product7/1(Out1) -> Product7_outbuff/1
  Product6/1(Out1) -> Product6_outbuff/1
  Data Type Conversion1/1(Out1) -> Goto35/1
  Data Type Conversion41/1(Out1) -> Goto33/1
  Data Type Conversion71/1(Out1) -> Goto10/1
  Data Type Conversion31/1(Out1) -> Goto34/1
  Product10/1(Out1) -> Product10_outbuff/1
  Product2/1(Out1) -> Product_outbuff/1
  Sum38/1(Out1) -> Sum3_outbuff8/1
  Sum1_stage2/1(Out1) -> Sum1_stage2_outbuff/1
  Sum1_stage3/1(Out1) -> Sum1_stage3_outbuff/1
  Data Type Conversion81/1(Out1) -> t5/1
  Data Type Conversion61/1(Out1) -> Switch2/1
  Data Type Conversion101/1(Out1) -> Switch2/3
  Add1/1(Out1) -> Add1_outbuff/1
  Divide2/1(Out1) -> Divide2_outbuff/1
  Divide3/1(Out1) -> Divide3_outbuff/1
  Sum39/1(Out1) -> Sum3_outbuff9/1
  Sum_stage2/1(Out1) -> Sum_stage2_outbuff/1
  Sum_stage3/1(Out1) -> Sum_stage3_outbuff/1
  Product8/1(Out1) -> Product8_outbuff/1
  Product5/1(Out1) -> Product5_outbuff/1
  Sum21/1(Out1) -> Sum2_outbuff1/1
  Product3/1(Out1) -> Product3_outbuff/1
  Product21/1(Out1) -> Product2_outbuff/1
  Sum310/1(Out1) -> Sum3_outbuff10/1
  Product9/1(Out1) -> Product9_outbuff/1
  Data Type Conversion15/1(Out1) -> Goto361/1
  Gain/1(Out1) -> Gain_outbuff/1
  Gain1/1(Out1) -> Gain_outbuff1/1
  Gain2/1(Out1) -> Sum/2(In2)
  Gain3/1(Out1) -> Gain_outbuff2/1
  Gain4/1(Out1) -> Gain_outbuff3/1
  Gain5/1(Out1) -> Gain_outbuff4/1
  Gain6/1(Out1) -> Gain_outbuff5/1
  Gain7/1(Out1) -> Gain_outbuff6/1
  Gain8/1(Out1) -> Gain_outbuff7/1
  Gain9/1(Out1) -> Gain_outbuff8/1
  Gain10/1(Out1) -> Gain_outbuff9/1
  Factor/1(Out1) -> Factor_outbuff/1
  delayMatch14/1 -> Product2/2(In2)
  delayMatch19/1 -> Product1/2(In2)
  From10/1 -> Product5/1(In1)
  pmsm_out1/1 -> delayMatch2/1
  pmsm_out2/1 -> delayMatch3/1
  Product3_outbuff/1 -> Sum310/1(In1)
  From41/1 -> Product9/2(In2)
  psi_/1 -> delayMatch4/1
  psi_6/1 -> delayMatch5/1
  psi_5/1 -> delayMatch6/1
  psi_4/1 -> delayMatch7/1
  psi_3/1 -> delayMatch8/1
  psi_2/1 -> delayMatch9/1
  psi_1/1 -> delayMatch10/1
  i_q/1 -> Product3/2(In2), mux/2
  mechanical_system_out1/1 -> delayMatch12/1
  From9/1 -> Product8/2(In2)
  psi_q/1 -> delayMatch14/1, delayMatch/1, pmsm_out2/1
  Product_outbuff/1 -> Sum_stage3/2(In2)
  reset_out10/1 -> delayMatch15/1, psi_d/1
  From25/1 -> delayMatch16/1, reset_out10/2
  From8/1 -> Divide2/1(In1)
  reset_out9/1 -> delayMatch17/1, psi_6/1
  From91/1 -> delayMatch18/1, reset_out9/2
  psi_d/1 -> delayMatch19/1, delayMatch1/1, pmsm_out1/1
  From12/1 -> Product7/2(In2)
  Product7_outbuff/1 -> Sum1_stage3/2(In2)
  reset_out8/1 -> delayMatch20/1, psi_q/1
  From32/1 -> delayMatch21/1, reset_out8/2
  reset_out1/1 -> delayMatch22/1, theta_el/1
  Compare To Constant_relop_outbuff/1 -> Switch/2
  Sum_outbuff/1 -> Compare To Constant_relop/1(In1), Sum11/1(In1), Switch/3
  Compare To Constant1_relop_outbuff/1 -> Switch1/2
  Switch/1 -> Sum2/2(In2), Compare To Constant1_relop/1(In1), Switch1/3
  From3/1 -> delayMatch23/1, reset_out1/2
  From1/1 -> Product11/1(In1)
  reset_out/1 -> delayMatch25/1, integrator_out1/1
  From2/1 -> delayMatch26/1, reset_out/2
  From4/1 -> Divide/1(In1)
  reset_out2/1 -> delayMatch27/1, psi_/1
  From5/1 -> delayMatch28/1, reset_out2/2
  From30/1 -> Divide12/1(In1)
  reset_out3/1 -> delayMatch29/1, psi_1/1
  From31/1 -> delayMatch30/1, reset_out3/2
  From26/1 -> Divide10/1(In1)
  reset_out4/1 -> delayMatch31/1, psi_2/1
  From27/1 -> delayMatch32/1, reset_out4/2
  From22/1 -> Divide8/1(In1)
  reset_out5/1 -> delayMatch33/1, psi_3/1
  From23/1 -> delayMatch34/1, reset_out5/2
  From18/1 -> Divide6/1(In1)
  reset_out6/1 -> delayMatch35/1, psi_4/1
  From19/1 -> delayMatch36/1, reset_out6/2
  From14/1 -> Divide4/1(In1)
  reset_out7/1 -> delayMatch37/1, psi_5/1
  From15/1 -> delayMatch38/1, reset_out7/2

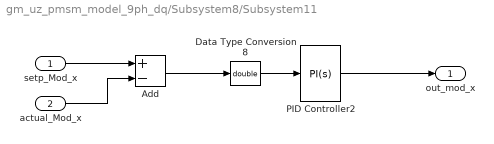
== system gm_uz_pmsm_model_9ph_dq/Subsystem8/Subsystem11 ==
  setp_Mod_x : Inport
  actual_Mod_x : Inport  Port=2
  Add : Sum  Inputs=+-
  Data Type Conversion8 : DataTypeConversion  OutDataTypeStr=double
  PID Controller2 : pid_lib/PID Controller  Controller=PI  Form=Ideal  TimeDomain=Continuous-time  UseExternalTs=off  SampleTime=-1  IntegratorMethod=Forward Euler  FilterMethod=Forward Euler  ControllerParametersSource=internal  P=Kpd  I=1/Tnd  D=0  N=100  UseFilter=on  TunerSelectOption=Transfer Function Based (PID Tuner App)  InitialConditionSource=internal  InitialConditionForIntegrator=0  InitialConditionForFilter=0  DifferentiatorICPrevScaledInput=0  ExternalReset=none  TrackingMode=off  Kt=1  LimitOutput=on  SatLimitsSource=internal  UpperSaturationLimit=50  LowerSaturationLimit=-50  LinearizeAsGain=on  AntiWindupMode=clamping  Kb=1  POutMin=[]  POutMax=[]  IOutMin=[]  IOutMax=[]  DOutMin=[]  DOutMax=[]  NOutMin=[]  NOutMax=[]  SumOutMin=[]  SumOutMax=[]  SaturationOutMin=[]  SaturationOutMax=[]  PParamMin=[]  PParamMax=[]  IParamMin=[]  IParamMax=[]  DParamMin=[]  DParamMax=[]  NParamMin=[]  NParamMax=[]  KbParamMin=[]  KbParamMax=[]  KtParamMin=[]  KtParamMax=[]  KbOutMin=[]  KbOutMax=[]  KtOutMin=[]  KtOutMax=[]  IntegratorOutMin=[]  IntegratorOutMax=[]  FilterOutMin=[]  FilterOutMax=[]  SumI1OutMin=[]  SumI1OutMax=[]  SumI2OutMin=[]  SumI2OutMax=[]  SumI3OutMin=[]  SumI3OutMax=[]  SumI4OutMin=[]  SumI4OutMax=[]  SumDOutMin=[]  SumDOutMax=[]  DifferentiatorOutMin=[]  DifferentiatorOutMax=[]  FilterDiffOutCoefMin=[]  FilterDiffOutCoefMax=[]  ReciprocalOutMin=[]  ReciprocalOutMax=[]  SumDenOutMin=[]  SumDenOutMax=[]  SumNumOutMin=[]  SumNumOutMax=[]  DivideOutMin=[]  DivideOutMax=[]  UdiffTsProdOutMin=[]  UdiffTsProdOutMax=[]  NTsProdOutMin=[]  NTsProdOutMax=[]  UintegralTsProdOutMin=[]  UintegralTsProdOutMax=[]  UngainTsProdOutMin=[]  UngainTsProdOutMax=[]  IntegratorContinuousStateAttributes=''  IntegratorStateMustResolveToSignalObject=off  IntegratorRTWStateStorageClass=Auto  FilterContinuousStateAttributes=''  FilterStateMustResolveToSignalObject=off  FilterRTWStateStorageClass=Auto  ParallelPVariant=Passthrough  IdealPVariant=InternalParameters  IVariant=InternalParameters  DVariant=Disabled  IntegratorVariant=Continuous  SatVariant=Enabled  AWVariant=ContClampingIdeal  PCopyVariant=InternalParamsIdeal  TRVariant=Disabled  FdbkBlocksVariant=Forward  IdealPFdbkVariant=Disabled  SatFdbkVariant=Disabled  DerivativeFilterVariant=Disabled  NVariant=Disabled  NCopyVariant=Disabled_SignalSpec  FilterICVariant=Disabled  IntegratorICVariant=InternalICs  ExternalResetVariant=Disabled  TRSumVariant=Passthrough  SumFdbkVariant=Disabled  SumVariant=Sum_PI  TsampFilterVariant=InternalTs  TsampNgainVariant=Passthrough  TsampIntegralVariant=Passthrough  ExternalSaturationOutDataTypeStr=Inherit: Same as second input
  out_mod_x : Outport
  wires:
  PID Controller2/1 -> out_mod_x/1
  setp_Mod_x/1 -> Add/1
  Data Type Conversion8/1 -> PID Controller2/1
  actual_Mod_x/1 -> Add/2
  Add/1 -> Data Type Conversion8/1

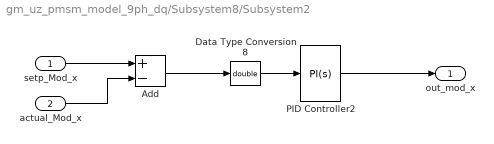
== system gm_uz_pmsm_model_9ph_dq/Subsystem8/Subsystem2 ==
  setp_Mod_x : Inport
  actual_Mod_x : Inport  Port=2
  Add : Sum  Inputs=+-
  Data Type Conversion8 : DataTypeConversion  OutDataTypeStr=double
  PID Controller2 : slpidlib/PID Controller  Controller=PI  Form=Ideal  TimeDomain=Continuous-time  UseExternalTs=off  SampleTime=-1  IntegratorMethod=Forward Euler  FilterMethod=Forward Euler  ControllerParametersSource=internal  P=k_p_d  I=k_i_d  D=0  UseFilter=on  N=100  TunerSelectOption=Transfer Function Based (PID Tuner App)  InitialConditionSource=internal  InitialConditionForIntegrator=0  InitialConditionForFilter=0  DifferentiatorICPrevScaledInput=0  ExternalReset=none  TrackingMode=off  Kt=1  LimitOutput=on  SatLimitsSource=internal  UpperSaturationLimit=100  LowerSaturationLimit=-100  LinearizeAsGain=on  AntiWindupMode=clamping  Kb=1  POutMin=[]  POutMax=[]  IOutMin=[]  IOutMax=[]  DOutMin=[]  DOutMax=[]  NOutMin=[]  NOutMax=[]  SumOutMin=[]  SumOutMax=[]  SaturationOutMin=[]  SaturationOutMax=[]  PParamMin=[]  PParamMax=[]  IParamMin=[]  IParamMax=[]  DParamMin=[]  DParamMax=[]  NParamMin=[]  NParamMax=[]  KbParamMin=[]  KbParamMax=[]  KtParamMin=[]  KtParamMax=[]  KbOutMin=[]  KbOutMax=[]  KtOutMin=[]  KtOutMax=[]  IntegratorOutMin=[]  IntegratorOutMax=[]  FilterOutMin=[]  FilterOutMax=[]  SumI1OutMin=[]  SumI1OutMax=[]  SumI2OutMin=[]  SumI2OutMax=[]  SumI3OutMin=[]  SumI3OutMax=[]  SumI4OutMin=[]  SumI4OutMax=[]  SumDOutMin=[]  SumDOutMax=[]  DifferentiatorOutMin=[]  DifferentiatorOutMax=[]  FilterDiffOutCoefMin=[]  FilterDiffOutCoefMax=[]  ReciprocalOutMin=[]  ReciprocalOutMax=[]  SumDenOutMin=[]  SumDenOutMax=[]  SumNumOutMin=[]  SumNumOutMax=[]  DivideOutMin=[]  DivideOutMax=[]  UdiffTsProdOutMin=[]  UdiffTsProdOutMax=[]  NTsProdOutMin=[]  NTsProdOutMax=[]  UintegralTsProdOutMin=[]  UintegralTsProdOutMax=[]  UngainTsProdOutMin=[]  UngainTsProdOutMax=[]  IntegratorContinuousStateAttributes=''  IntegratorStateMustResolveToSignalObject=off  IntegratorRTWStateStorageClass=Auto  FilterContinuousStateAttributes=''  FilterStateMustResolveToSignalObject=off  FilterRTWStateStorageClass=Auto  ParallelPVariant=Passthrough  IdealPVariant=InternalParameters  IVariant=InternalParameters  DVariant=Disabled  IntegratorVariant=Continuous  SatVariant=Enabled  AWVariant=ContClampingIdeal  PCopyVariant=InternalParamsIdeal  TRVariant=Disabled  FdbkBlocksVariant=Forward  IdealPFdbkVariant=Disabled  SatFdbkVariant=Disabled  DerivativeFilterVariant=Disabled  NVariant=Disabled  NCopyVariant=Disabled_SignalSpec  FilterICVariant=Disabled  IntegratorICVariant=InternalICs  ExternalResetVariant=Disabled  TRSumVariant=Passthrough  SumFdbkVariant=Disabled  SumVariant=Sum_PI  TsampFilterVariant=InternalTs  TsampNgainVariant=Passthrough  TsampIntegralVariant=Passthrough  ExternalSaturationOutDataTypeStr=Inherit: Same as second input
  out_mod_x : Outport
  wires:
  PID Controller2/1 -> out_mod_x/1
  setp_Mod_x/1 -> Add/1
  Data Type Conversion8/1 -> PID Controller2/1
  actual_Mod_x/1 -> Add/2
  Add/1 -> Data Type Conversion8/1
